simulink model "EEL_5661_F21_Bicycle_OL_091521"  (R2019a)
settings: Solver=VariableStepAuto  StartTime=0.0  StopTime=4  RelTol=1e-3
libraries: simulink x1
settings Model: Creator=rothz  LastModifiedBy=rothz

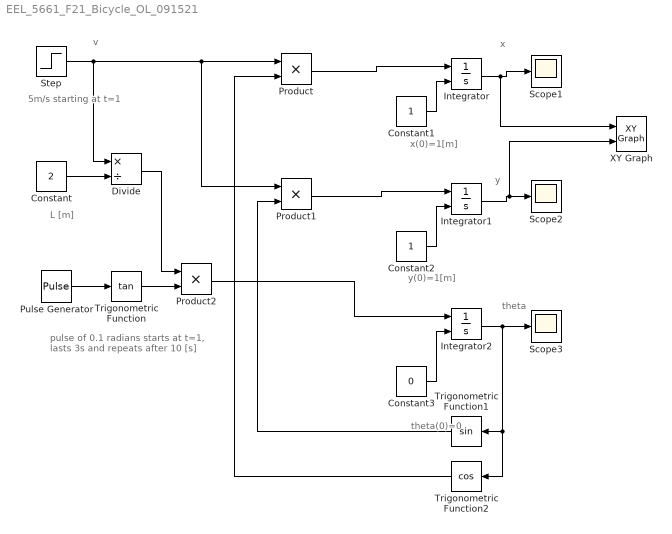
== system EEL_5661_F21_Bicycle_OL_091521 ==
  note: pulse of 0.1 radians starts
      | at t=1, lasts 3s and repeats after
      | 10 [s]
  note: theta(0)=0
  note: y(0)=1[m]
  note: x(0)=1[m]
  note: L [m]
  note: 5m/s starting at t=1
  note: v
  note: theta
  note: y
  note: x
  Constant : Constant  Value=2
  Constant1 : Constant
  Constant2 : Constant
  Constant3 : Constant  Value=0
  Divide : Product  Inputs=*/
  Integrator : Integrator  InitialConditionSource=external
  Integrator1 : Integrator  InitialConditionSource=external
  Integrator2 : Integrator  InitialConditionSource=external
  Product : Product
  Product1 : Product
  Product2 : Product
  Pulse Generator : DiscretePulseGenerator  PulseType=Time based  Amplitude=0.1  Period=10  PulseWidth=30  PhaseDelay=1
  Scope1 : Scope
  Scope2 : Scope
  Scope3 : Scope
  Step : Step  After=5  SampleTime=0
  Trigonometric Function : Trigonometry  Operator=tan
  Trigonometric Function1 : Trigonometry
  Trigonometric Function2 : Trigonometry  Operator=cos
  XY Graph : simulink/Sinks/XY Graph  xmin=-1  xmax=20  ymin=-1  ymax=20  st=-1
  wires:
  Integrator2/1 -> Trigonometric Function2/1, Trigonometric Function1/1, Scope3/1
  Step/1 -> Divide/1, Product1/1, Product/1
  Trigonometric Function1/1 -> Product1/2
  Trigonometric Function2/1 -> Product/2
  Constant/1 -> Divide/2
  Divide/1 -> Product2/1
  Pulse Generator/1 -> Trigonometric Function/1
  Trigonometric Function/1 -> Product2/2
  Product2/1 -> Integrator2/1
  Constant3/1 -> Integrator2/2
  Constant2/1 -> Integrator1/2
  Product1/1 -> Integrator1/1
  Constant1/1 -> Integrator/2
  Product/1 -> Integrator/1
  Integrator/1 -> XY Graph/1, Scope1/1
  Integrator1/1 -> XY Graph/2, Scope2/1
